simulink model "Q1_arthamatic_stateflow"  (R2024b)
settings: Solver=VariableStepAuto  StartTime=0.0  StopTime=10.0  RelTol=1e-3
model workspace (MAT data in the model file):
  choice = 2
settings Model: Creator=chall  LastModifiedBy=chall

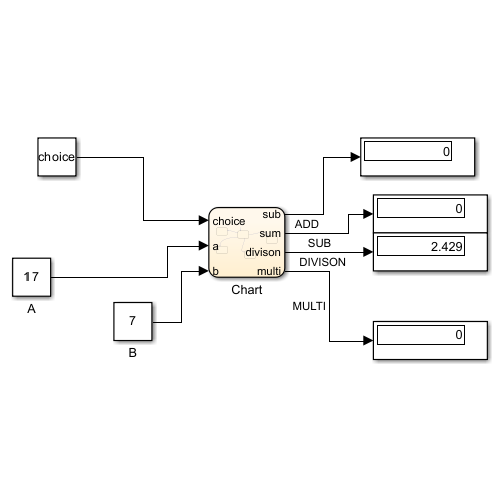
[thumbnail: Simulink's stored preview of the top-level diagram]
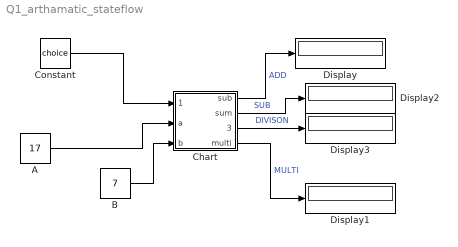
== system Q1_arthamatic_stateflow ==
  A : Constant  Value=17
  B : Constant  Value=7
  Chart : Stateflow chart  TreatAsAtomicUnit=on
  Constant : Constant  Value=choice
  Display{,1..3} (4 alike) : Display
  wires:
  Constant/1 -> Chart/1(choice)
  B/1 -> Chart/3(b)
  A/1 -> Chart/2(a)
  Chart/1(sub) -> Display/1  "ADD"
  Chart/4(multi) -> Display1/1  "MULTI"
  Chart/2(sum) -> Display2/1  "SUB"
  Chart/3(divison) -> Display3/1  "DIVISON"

== stateflow chart Q1_arthamatic_stateflow/Chart ==
  state addition
    entry :
    sum =a+b ;
  state choice
  state division
    entry:
    divison = a/b;
  state subtraction
    entry:
    sub = a-b;
  state multipication
    entry:
    multi =a*b
  (default) -> choice
  choice -> addition [order 1] : [choice ==1]
  choice -> division [order 4] : [choice ==4]
  choice -> subtraction [order 3] : [choice ==2]
  choice -> multipication [order 2] : [choice ==3]
  data: choice input; a input; b input; sub output; sum output; divison output; multi output
